simulink model "k1visbsp"  (Simulink 8.8)
settings: Solver=ode45  StartTime=0.0  StopTime=10.0  RelTol=1e-3  EnableMultiTasking=on
libraries: cdsIPCx x16, cdsEpicsOut x7, cdsBit2Word x6, cdsEpicsBinIn x3, cdsWord2Bit x3, cdsCDI64 x3, cdsCDO64 x3, TYPEB_MASTER x2, dac x2, cdsAdcx0 x1, cdsParameters x1
settings Model: SuppressorTable=22 serialization::archive 11 0 3 0 0 0 11 0  Creator=controls  LastModifiedBy=controls
settings DataIOCC: SignalLoggingSaveFormat=Dataset
settings DebuggingCC: UnderspecifiedInitializationDetection=Simplified  MergeDetectMultiDrivingBlocksExec=error  FcnCallInpInsideContextMsg=error  AllowSymbolicDim=off  StateNameClashWarn=none
settings GRTTargetCC: CombineOutputUpdateFcns=on  GRTInterface=off

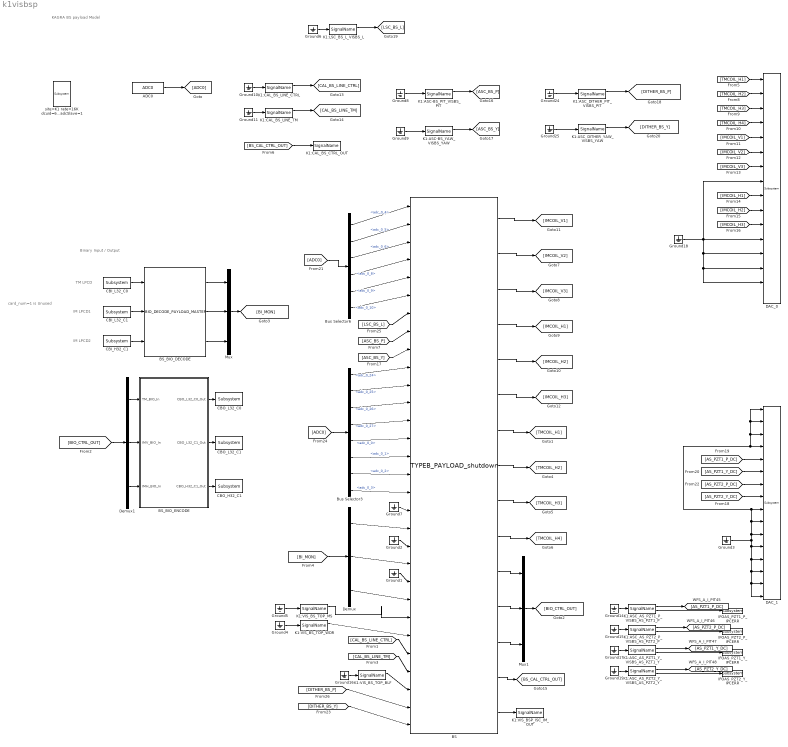
== system k1visbsp ==
  note: KAGRA BS payload Model
  note: TM LPCD
  note: Binary Input / Output
  note: card_num=1 is Unused
  note: IM LPCD1
  note: IM LPCD2
  ADC0 : cdsAdcx0/ADC0  Tag=cdsAdc  Description=|
      | type-GSC_16AI64SSA
      | card_num=0
      settings: AttributesFormatString=%<Description>\n%<Tag>
  BS : TYPEB_MASTER/TYPEB_PAYLOAD_shutdown
  BS_BIO_DECODE : TYPEB_MASTER/BIO_DECODE_PAYLOAD_MASTER
  BS_BIO_ENCODE : Subsystem  AncestorBlock=TYPEB_MASTER/BIO_ENCODE_PAYLOAD_MASTER
  Bus Selector3 : BusSelector  Description=ADC Selector  OutputSignals=adc_0_24,adc_0_25,adc_0_26,adc_0_27,adc_0_0,adc_0_1,adc_0_2,adc_0_3
      settings: AttributesFormatString=%<Description>
  Bus Selector6 : BusSelector  Description=ADC Selector  OutputSignals=adc_0_4,adc_0_5,adc_0_6,adc_0_8,adc_0_9,adc_0_10
      settings: AttributesFormatString=%<Description>
  CBI_H32_C1 : cdsCDI64/Subsystem  Tag=cdsCDI64  Description=card_num=3
      settings: AttributesFormatString=%<Tag>\n%<Description>
  CBI_L32_C0 : cdsCDI64/Subsystem  Tag=cdsCDI64  Description=card_num=0
      settings: AttributesFormatString=%<Tag>\n%<Description>
  CBI_L32_C1 : cdsCDI64/Subsystem  Tag=cdsCDI64  Description=card_num=2
      settings: AttributesFormatString=%<Tag>\n%<Description>
  CBO_H32_C1 : cdsCDO64/Subsystem  Tag=cdsCDO64  Description=card_num=3
      settings: AttributesFormatString=%<Tag>\n%<Description>
  CBO_L32_C0 : cdsCDO64/Subsystem  Tag=cdsCDO64  Description=card_num=0
      settings: AttributesFormatString=%<Tag>\n%<Description>
  CBO_L32_C1 : cdsCDO64/Subsystem  Tag=cdsCDO64  Description=card_num=2
      settings: AttributesFormatString=%<Tag>\n%<Description>
  DAC_0 : dac/Subsystem  Description=|
      | type=GSC_16AO16,
      | card_num=0
      settings: AttributesFormatString=%<Description>
  DAC_1 : dac/Subsystem  Description=|
      | type=GSC_16AO16,
      | card_num=1
      settings: AttributesFormatString=%<Description>
  Demux : Demux  Outputs=3
  Demux1 : Demux  Outputs=3
  Ground{1..11,14..19,24..25} (19 alike) : Ground
  IFOAS_PZT1_P_IPCERR : cdsEpicsOut/Subsystem  Tag=cdsEpicsOutput  Description=|
      | Purpose:                                          
      | Output a FE signal to an EPICS channel.           
      |                                                   
      | Operation:                                        
      | Takes input value and passes it to EPICS record.  
      |                                                   
      | Usage:                                            
      | Name the part with the desired EPICS rrecord name.
      settings: AttributesFormatString=%<Tag>
  IFOAS_PZT1_Y_IPCERR : cdsEpicsOut/Subsystem  Tag=cdsEpicsOutput  Description=|
      | Purpose:                                          
      | Output a FE signal to an EPICS channel.           
      |                                                   
      | Operation:                                        
      | Takes input value and passes it to EPICS record.  
      |                                                   
      | Usage:                                            
      | Name the part with the desired EPICS rrecord name.
      settings: AttributesFormatString=%<Tag>
  IFOAS_PZT2_P_IPCERR : cdsEpicsOut/Subsystem  Tag=cdsEpicsOutput  Description=|
      | Purpose:                                          
      | Output a FE signal to an EPICS channel.           
      |                                                   
      | Operation:                                        
      | Takes input value and passes it to EPICS record.  
      |                                                   
      | Usage:                                            
      | Name the part with the desired EPICS rrecord name.
      settings: AttributesFormatString=%<Tag>
  IFOAS_PZT2_Y_IPCERR : cdsEpicsOut/Subsystem  Tag=cdsEpicsOutput  Description=|
      | Purpose:                                          
      | Output a FE signal to an EPICS channel.           
      |                                                   
      | Operation:                                        
      | Takes input value and passes it to EPICS record.  
      |                                                   
      | Usage:                                            
      | Name the part with the desired EPICS rrecord name.
      settings: AttributesFormatString=%<Tag>
  K1:ASC-BS_PIT_VISBS_PIT : cdsIPCx/SignalName  Tag=cdsIPCx_PCIE  Description=Inter-Process Communication via PCI Express network.
      settings: AttributesFormatString=%<Tag>
  K1:ASC-BS_YAW_VISBS_YAW : cdsIPCx/SignalName  Tag=cdsIPCx_PCIE  Description=Inter-Process Communication via PCI Express network.
      settings: AttributesFormatString=%<Tag>
  K1:ASC_AS_PZT1_P_VISBS_AS_PZT1_P : cdsIPCx/SignalName  Tag=cdsIPCx_PCIE  Description=Inter-Process Communication via PCI Express network.
      settings: AttributesFormatString=%<Tag>
  K1:ASC_AS_PZT1_Y_VISBS_AS_PZT1_Y : cdsIPCx/SignalName  Tag=cdsIPCx_PCIE  Description=Inter-Process Communication via PCI Express network.
      settings: AttributesFormatString=%<Tag>
  K1:ASC_AS_PZT2_P_VISBS_AS_PZT2_P : cdsIPCx/SignalName  Tag=cdsIPCx_PCIE  Description=Inter-Process Communication via PCI Express network.
      settings: AttributesFormatString=%<Tag>
  K1:ASC_AS_PZT2_Y_VISBS_AS_PZT2_Y : cdsIPCx/SignalName  Tag=cdsIPCx_PCIE  Description=Inter-Process Communication via PCI Express network.
      settings: AttributesFormatString=%<Tag>
  K1:ASC_DITHER_PIT_VISBS_PIT : cdsIPCx/SignalName  Tag=cdsIPCx_PCIE  Description=Inter-Process Communication via PCI Express network.
      settings: AttributesFormatString=%<Tag>
  K1:ASC_DITHER_YAW_VISBS_YAW : cdsIPCx/SignalName  Tag=cdsIPCx_PCIE  Description=Inter-Process Communication via PCI Express network.
      settings: AttributesFormatString=%<Tag>
  K1:CAL_BS_CTRL_OUT : cdsIPCx/SignalName  Tag=cdsIPCx_PCIE  Description=Inter-Process Communication via PCI Express network.
      settings: AttributesFormatString=%<Tag>
  K1:CAL_BS_LINE_CTRL : cdsIPCx/SignalName  Tag=cdsIPCx_PCIE  Description=Inter-Process Communication via PCI Express network.
      settings: AttributesFormatString=%<Tag>
  K1:CAL_BS_LINE_TM : cdsIPCx/SignalName  Tag=cdsIPCx_PCIE  Description=Inter-Process Communication via PCI Express network.
      settings: AttributesFormatString=%<Tag>
  K1:LSC_BS_L_VISBS_L : cdsIPCx/SignalName  Tag=cdsIPCx_PCIE  Description=Inter-Process Communication via PCI Express network.
      settings: AttributesFormatString=%<Tag>
  K1:VIS_BSP_ISC_IM_OUT : cdsIPCx/SignalName  Tag=cdsIPCx_SHMEM  Description=Inter-Process Communication via Shared memory.
      settings: AttributesFormatString=%<Tag>
  K1:VIS_BS_TOP_BLF : cdsIPCx/SignalName  Tag=cdsIPCx_SHMEM  Description=Inter-Process Communication via Shared memory.
      settings: AttributesFormatString=%<Tag>
  K1:VIS_BS_TOP_MS : cdsIPCx/SignalName  Tag=cdsIPCx_SHMEM  Description=Inter-Process Communication via Shared memory.
      settings: AttributesFormatString=%<Tag>
  K1:VIS_BS_TOP_WDR : cdsIPCx/SignalName  Tag=cdsIPCx_SHMEM  Description=Inter-Process Communication via Shared memory.
      settings: AttributesFormatString=%<Tag>
  Mux : Mux  Inputs=3
  Mux1 : Mux  Inputs=3
  site=K1 rate=16K dcuid=61 host=k1bs specific_cpu=3 adcSlave=1 : cdsParameters/Subsystem  Tag=cdsParameters  Description=|
      | Purpose:                                                                                                                                                                                                                                
      | Provide system parameters to the FE code generator to properly configure the generated EPICS names, rep rate of the FE controller, and the Data Acquisition node ID for proper storage of data from this FE controller.                 
      |                                                                                                                                                                                                                                         
      | Useage:                                                                                                                                                                                                                                 
      | The part NAME field is used to identify the FE parameters. It must be of the form:                                                                                                                                                      
      | site=                                                                                                                                                                                                                                   
      | rate=                                                                                                                                                                                                                                   
      | dcuid=                                                                                                                                                                                                                                  
      |                                                                                                                                                                                                                                         
      | Where:                                                                                                                                                                                                                                  
      | site= argument may be H1, H2, L1, M1, G1, either as a single argument or multiple, for example site=H1,H2. These are the only names allowed. These will become the first two characters of all EPICS and signal names (for example G1:).
      |                                                                                                                                                                                                                                         
      | rate= may be 2K, 16K, 32K, or 64K                                                                                                                                                                                                       
      |                                                                                                                                                                                                                                         
      | dcuid= is site specific ie it must be unique at each site.
      settings: AttributesFormatString=%<Tag>
  wires:
  ADC0/1 -> [ADC0]
  [ADC0] -> Bus Selector6/1
  BS/10 -> [TMCOIL_H4]
  BS/9 -> [TMCOIL_H3]
  BS/8 -> [TMCOIL_H2]
  BS/7 -> [TMCOIL_H1]
  BS/1 -> [IMCOIL_V1]
  BS/2 -> [IMCOIL_V2]
  BS/3 -> [IMCOIL_V3]
  BS/4 -> [IMCOIL_H1]
  BS/5 -> [IMCOIL_H2]
  BS/6 -> [IMCOIL_H3]
  Ground18/1 -> DAC_0/12, DAC_0/13, DAC_0/14, DAC_0/15, DAC_0/8
  Bus Selector6/1 -> BS/1  "<adc_0_4>"
  Bus Selector6/2 -> BS/2  "<adc_0_5>"
  Bus Selector6/3 -> BS/3  "<adc_0_6>"
  [TMCOIL_H2] -> DAC_0/2
  [TMCOIL_H3] -> DAC_0/3
  [TMCOIL_H1] -> DAC_0/1
  [TMCOIL_H4] -> DAC_0/4
  [IMCOIL_V1] -> DAC_0/5
  [IMCOIL_V2] -> DAC_0/6
  [IMCOIL_V3] -> DAC_0/7
  Bus Selector6/4 -> BS/4  "<adc_0_8>"
  Bus Selector6/5 -> BS/5  "<adc_0_9>"
  Bus Selector6/6 -> BS/6  "<adc_0_10>"
  [IMCOIL_H3] -> DAC_0/11
  [IMCOIL_H2] -> DAC_0/10
  [IMCOIL_H1] -> DAC_0/9
  [LSC_BS_L] -> BS/7
  [ADC0] -> Bus Selector3/1
  Bus Selector3/1 -> BS/10  "<adc_0_24>"
  Bus Selector3/2 -> BS/11  "<adc_0_25>"
  Bus Selector3/3 -> BS/12  "<adc_0_26>"
  Bus Selector3/4 -> BS/13  "<adc_0_27>"
  BS_BIO_ENCODE/3(CBO_H32_C1_Out) -> CBO_H32_C1/1
  BS_BIO_ENCODE/2(CBO_L32_C1_Out) -> CBO_L32_C1/1
  CBI_L32_C1/1 -> BS_BIO_DECODE/2
  CBI_H32_C1/1 -> BS_BIO_DECODE/3
  BS_BIO_DECODE/2 -> Mux/2
  BS_BIO_DECODE/3 -> Mux/3
  BS_BIO_DECODE/1 -> Mux/1
  Mux/1 -> [BI_MON]
  Demux1/2 -> BS_BIO_ENCODE/2(IMV_BIO_In)
  Demux1/3 -> BS_BIO_ENCODE/3(IMH_BIO_In)
  Demux1/1 -> BS_BIO_ENCODE/1(TM_BIO_In)
  [BIO_CTRL_OUT] -> Demux1/1
  Mux1/1 -> [BIO_CTRL_OUT]
  [BI_MON] -> Demux/1
  Demux/1 -> BS/19
  Demux/2 -> BS/21
  Demux/3 -> BS/23
  Ground7/1 -> BS/18
  Ground1/1 -> BS/22
  Ground2/1 -> BS/20
  Ground4/1 -> K1:VIS_BS_TOP_WDR/1
  Ground5/1 -> K1:VIS_BS_TOP_MS/1
  K1:VIS_BS_TOP_WDR/1 -> BS/25
  K1:VIS_BS_TOP_MS/1 -> BS/24
  Ground10/1 -> K1:CAL_BS_LINE_CTRL/1
  K1:CAL_BS_LINE_CTRL/1 -> [CAL_BS_LINE_CTRL]
  Ground11/1 -> K1:CAL_BS_LINE_TM/1
  K1:CAL_BS_LINE_TM/1 -> [CAL_BS_LINE_TM]
  [CAL_BS_LINE_CTRL] -> BS/26
  [CAL_BS_LINE_TM] -> BS/27
  BS/14 -> [BS_CAL_CTRL_OUT]
  [BS_CAL_CTRL_OUT] -> K1:CAL_BS_CTRL_OUT/1
  Ground3/1 -> DAC_1/13, DAC_1/14, DAC_1/15, DAC_1/16, DAC_1/12, DAC_1/1, DAC_1/2, DAC_1/3, DAC_1/4, DAC_1/9, DAC_1/10, DAC_1/11
  Bus Selector3/5 -> BS/14  "<adc_0_0>"
  Bus Selector3/6 -> BS/15  "<adc_0_1>"
  Bus Selector3/7 -> BS/16  "<adc_0_2>"
  Bus Selector3/8 -> BS/17  "<adc_0_3>"
  [ASC_BS_P] -> BS/8
  [ASC_BS_Y] -> BS/9
  Ground16/1 -> K1:VIS_BS_TOP_BLF/1
  K1:VIS_BS_TOP_BLF/1 -> BS/28
  BS/11 -> Mux1/1
  BS/12 -> Mux1/2
  BS/13 -> Mux1/3
  [DITHER_BS_Y] -> BS/30
  K1:ASC_AS_PZT1_P_VISBS_AS_PZT1_P/2 -> IFOAS_PZT1_P_IPCERR/1
  K1:ASC_AS_PZT2_P_VISBS_AS_PZT2_P/2 -> IFOAS_PZT2_P_IPCERR/1
  K1:ASC_AS_PZT1_Y_VISBS_AS_PZT1_Y/2 -> IFOAS_PZT1_Y_IPCERR/1
  K1:ASC_AS_PZT2_Y_VISBS_AS_PZT2_Y/2 -> IFOAS_PZT2_Y_IPCERR/1
  K1:ASC_AS_PZT1_P_VISBS_AS_PZT1_P/1 -> [AS_PZT1_P_DC]
  K1:ASC_AS_PZT2_P_VISBS_AS_PZT2_P/1 -> [AS_PZT2_P_DC]
  K1:ASC_AS_PZT1_Y_VISBS_AS_PZT1_Y/1 -> [AS_PZT1_Y_DC]
  K1:ASC_AS_PZT2_Y_VISBS_AS_PZT2_Y/1 -> [AS_PZT2_Y_DC]
  Ground14/1 -> K1:ASC_AS_PZT1_P_VISBS_AS_PZT1_P/1
  Ground15/1 -> K1:ASC_AS_PZT2_P_VISBS_AS_PZT2_P/1
  Ground17/1 -> K1:ASC_AS_PZT1_Y_VISBS_AS_PZT1_Y/1
  Ground19/1 -> K1:ASC_AS_PZT2_Y_VISBS_AS_PZT2_Y/1
  [AS_PZT2_Y_DC] -> DAC_1/8
  [AS_PZT2_P_DC] -> DAC_1/7
  [AS_PZT1_Y_DC] -> DAC_1/6
  [AS_PZT1_P_DC] -> DAC_1/5
  Ground6/1 -> K1:LSC_BS_L_VISBS_L/1
  K1:LSC_BS_L_VISBS_L/1 -> [LSC_BS_L]
  Ground8/1 -> K1:ASC-BS_PIT_VISBS_PIT/1
  Ground9/1 -> K1:ASC-BS_YAW_VISBS_YAW/1
  Ground25/1 -> K1:ASC_DITHER_YAW_VISBS_YAW/1
  Ground24/1 -> K1:ASC_DITHER_PIT_VISBS_PIT/1
  [DITHER_BS_P] -> BS/29
  K1:ASC-BS_PIT_VISBS_PIT/1 -> [ASC_BS_P]
  K1:ASC-BS_YAW_VISBS_YAW/1 -> [ASC_BS_Y]
  K1:ASC_DITHER_PIT_VISBS_PIT/1 -> [DITHER_BS_P]
  K1:ASC_DITHER_YAW_VISBS_YAW/1 -> [DITHER_BS_Y]
  BS_BIO_ENCODE/1(CBO_L32_C0_Out) -> CBO_L32_C0/1
  CBI_L32_C0/1 -> BS_BIO_DECODE/1
  BS/15 -> K1:VIS_BSP_ISC_IM_OUT/1

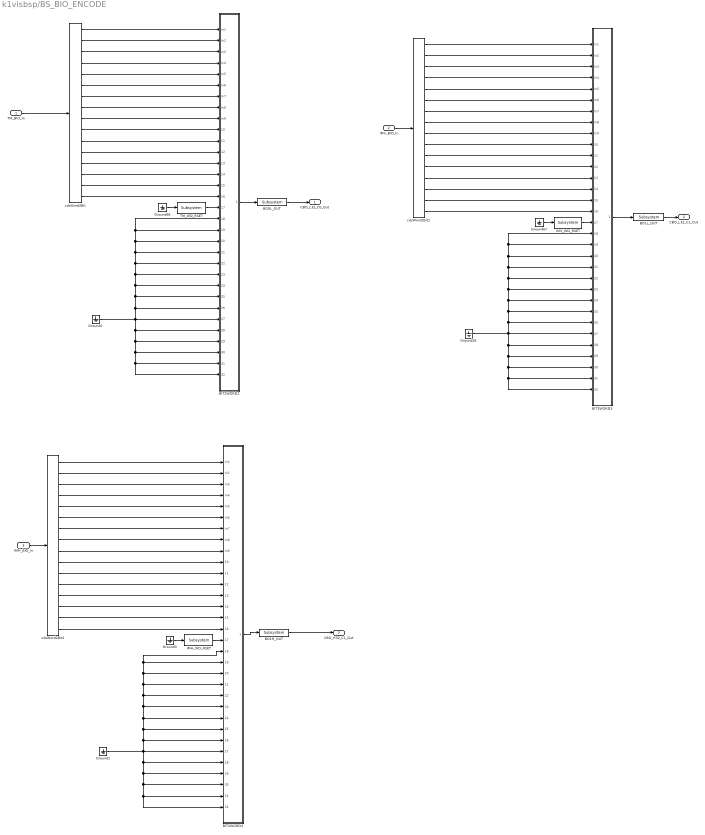
== system k1visbsp/BS_BIO_ENCODE ==
  TM_BIO_In : Inport
  IMV_BIO_In : Inport  Port=2
  IMH_BIO_In : Inport  Port=3
  BIT2WORD2 : Subsystem
  BIT2WORD3 : Subsystem
  BIT2WORD4 : Subsystem
  BO0L_OUT : cdsEpicsOut/Subsystem  Tag=cdsEpicsOutput  Description=|
      | Purpose:                                          
      | Output a FE signal to an EPICS channel.           
      |                                                   
      | Operation:                                        
      | Takes input value and passes it to EPICS record.  
      |                                                   
      | Usage:                                            
      | Name the part with the desired EPICS rrecord name.
      settings: AttributesFormatString=%<Tag>
  BO1H_OUT : cdsEpicsOut/Subsystem  Tag=cdsEpicsOutput  Description=|
      | Purpose:                                          
      | Output a FE signal to an EPICS channel.           
      |                                                   
      | Operation:                                        
      | Takes input value and passes it to EPICS record.  
      |                                                   
      | Usage:                                            
      | Name the part with the desired EPICS rrecord name.
      settings: AttributesFormatString=%<Tag>
  BO1L_OUT : cdsEpicsOut/Subsystem  Tag=cdsEpicsOutput  Description=|
      | Purpose:                                          
      | Output a FE signal to an EPICS channel.           
      |                                                   
      | Operation:                                        
      | Takes input value and passes it to EPICS record.  
      |                                                   
      | Usage:                                            
      | Name the part with the desired EPICS rrecord name.
      settings: AttributesFormatString=%<Tag>
  Ground{1..3,26,66..67} (6 alike) : Ground
  IMH_WD_RSET : cdsEpicsBinIn/Subsystem  Tag=cdsEpicsBinIn  Description=|
      | Purpose:                                                                            
      | Create an EPICS binary (0 or 1) input channel to the FE realtime controls.          
      |                                                                                     
      | Operation:                                                                          
      | Outputs value from an EPICS ai record. Value is binary input (bi Epics record type).
      |                                                                                     
      | Usage:                                                                              
      | Name the part with the desired EPICS channel name.
      settings: AttributesFormatString=%<Tag>
  IMV_WD_RSET : cdsEpicsBinIn/Subsystem  Tag=cdsEpicsBinIn  Description=|
      | Purpose:                                                                            
      | Create an EPICS binary (0 or 1) input channel to the FE realtime controls.          
      |                                                                                     
      | Operation:                                                                          
      | Outputs value from an EPICS ai record. Value is binary input (bi Epics record type).
      |                                                                                     
      | Usage:                                                                              
      | Name the part with the desired EPICS channel name.
      settings: AttributesFormatString=%<Tag>
  TM_WD_RSET : cdsEpicsBinIn/Subsystem  Tag=cdsEpicsBinIn  Description=|
      | Purpose:                                                                            
      | Create an EPICS binary (0 or 1) input channel to the FE realtime controls.          
      |                                                                                     
      | Operation:                                                                          
      | Outputs value from an EPICS ai record. Value is binary input (bi Epics record type).
      |                                                                                     
      | Usage:                                                                              
      | Name the part with the desired EPICS channel name.
      settings: AttributesFormatString=%<Tag>
  cdsWord2Bit : cdsWord2Bit/cdsWord2Bit  Tag=cdsWord2Bit  Description=Generate 16 0/1 outputs from single 16-bit integer input
      settings: AttributesFormatString=cdsWord2Bit
  cdsWord2Bit1 : cdsWord2Bit/cdsWord2Bit  Tag=cdsWord2Bit  Description=Generate 16 0/1 outputs from single 16-bit integer input
      settings: AttributesFormatString=cdsWord2Bit
  cdsWord2Bit2 : cdsWord2Bit/cdsWord2Bit  Tag=cdsWord2Bit  Description=Generate 16 0/1 outputs from single 16-bit integer input
      settings: AttributesFormatString=cdsWord2Bit
  CBO_L32_C0_Out : Outport
  CBO_L32_C1_Out : Outport  Port=2
  CBO_H32_C1_Out : Outport  Port=3
  wires:
  cdsWord2Bit2/16 -> BIT2WORD4/16(In16)
  cdsWord2Bit2/12 -> BIT2WORD4/12(In12)
  cdsWord2Bit2/14 -> BIT2WORD4/14(In14)
  cdsWord2Bit2/15 -> BIT2WORD4/15(In15)
  cdsWord2Bit2/13 -> BIT2WORD4/13(In13)
  cdsWord2Bit1/13 -> BIT2WORD3/13(In13)
  cdsWord2Bit1/15 -> BIT2WORD3/15(In15)
  cdsWord2Bit1/14 -> BIT2WORD3/14(In14)
  cdsWord2Bit1/16 -> BIT2WORD3/16(In16)
  cdsWord2Bit1/12 -> BIT2WORD3/12(In12)
  cdsWord2Bit/16 -> BIT2WORD2/16(In16)
  cdsWord2Bit/15 -> BIT2WORD2/15(In15)
  cdsWord2Bit/14 -> BIT2WORD2/14(In14)
  cdsWord2Bit/13 -> BIT2WORD2/13(In13)
  cdsWord2Bit/12 -> BIT2WORD2/12(In12)
  IMH_WD_RSET/1 -> BIT2WORD4/17(In17)
  Ground3/1 -> IMH_WD_RSET/1
  cdsWord2Bit2/11 -> BIT2WORD4/11(In11)
  cdsWord2Bit2/10 -> BIT2WORD4/10(In10)
  cdsWord2Bit2/9 -> BIT2WORD4/9(In9)
  cdsWord2Bit2/8 -> BIT2WORD4/8(In8)
  cdsWord2Bit2/7 -> BIT2WORD4/7(In7)
  cdsWord2Bit2/1 -> BIT2WORD4/1(In1)
  cdsWord2Bit2/6 -> BIT2WORD4/6(In6)
  cdsWord2Bit2/2 -> BIT2WORD4/2(In2)
  cdsWord2Bit2/3 -> BIT2WORD4/3(In3)
  cdsWord2Bit2/5 -> BIT2WORD4/5(In5)
  cdsWord2Bit2/4 -> BIT2WORD4/4(In4)
  IMH_BIO_In/1 -> cdsWord2Bit2/1
  Ground1/1 -> BIT2WORD4/31(In31), BIT2WORD4/32(In32), BIT2WORD4/30(In30), BIT2WORD4/29(In29), BIT2WORD4/28(In28), BIT2WORD4/18(In18), BIT2WORD4/19(In19), BIT2WORD4/20(In20), BIT2WORD4/21(In21), BIT2WORD4/22(In22), BIT2WORD4/23(In23), BIT2WORD4/24(In24), BIT2WORD4/25(In25), BIT2WORD4/26(In26), BIT2WORD4/27(In27)
  BIT2WORD4/1(Out1) -> BO1H_OUT/1
  BO1L_OUT/1 -> CBO_L32_C1_Out/1
  BIT2WORD3/1(Out1) -> BO1L_OUT/1
  BIT2WORD2/1(Out1) -> BO0L_OUT/1
  BO1H_OUT/1 -> CBO_H32_C1_Out/1
  BO0L_OUT/1 -> CBO_L32_C0_Out/1
  IMV_WD_RSET/1 -> BIT2WORD3/17(In17)
  TM_WD_RSET/1 -> BIT2WORD2/17(In17)
  Ground67/1 -> IMV_WD_RSET/1
  Ground66/1 -> TM_WD_RSET/1
  cdsWord2Bit1/11 -> BIT2WORD3/11(In11)
  cdsWord2Bit1/10 -> BIT2WORD3/10(In10)
  cdsWord2Bit1/9 -> BIT2WORD3/9(In9)
  cdsWord2Bit1/8 -> BIT2WORD3/8(In8)
  cdsWord2Bit1/7 -> BIT2WORD3/7(In7)
  cdsWord2Bit1/1 -> BIT2WORD3/1(In1)
  cdsWord2Bit1/6 -> BIT2WORD3/6(In6)
  cdsWord2Bit1/2 -> BIT2WORD3/2(In2)
  cdsWord2Bit1/3 -> BIT2WORD3/3(In3)
  cdsWord2Bit1/5 -> BIT2WORD3/5(In5)
  cdsWord2Bit1/4 -> BIT2WORD3/4(In4)
  IMV_BIO_In/1 -> cdsWord2Bit1/1
  Ground26/1 -> BIT2WORD3/27(In27), BIT2WORD3/29(In29), BIT2WORD3/30(In30), BIT2WORD3/32(In32), BIT2WORD3/31(In31), BIT2WORD3/28(In28), BIT2WORD3/26(In26), BIT2WORD3/25(In25), BIT2WORD3/24(In24), BIT2WORD3/23(In23), BIT2WORD3/22(In22), BIT2WORD3/21(In21), BIT2WORD3/19(In19), BIT2WORD3/18(In18), BIT2WORD3/20(In20)
  cdsWord2Bit/11 -> BIT2WORD2/11(In11)
  cdsWord2Bit/10 -> BIT2WORD2/10(In10)
  cdsWord2Bit/9 -> BIT2WORD2/9(In9)
  cdsWord2Bit/8 -> BIT2WORD2/8(In8)
  cdsWord2Bit/7 -> BIT2WORD2/7(In7)
  cdsWord2Bit/1 -> BIT2WORD2/1(In1)
  cdsWord2Bit/2 -> BIT2WORD2/2(In2)
  cdsWord2Bit/3 -> BIT2WORD2/3(In3)
  cdsWord2Bit/4 -> BIT2WORD2/4(In4)
  TM_BIO_In/1 -> cdsWord2Bit/1
  Ground2/1 -> BIT2WORD2/27(In27), BIT2WORD2/29(In29), BIT2WORD2/30(In30), BIT2WORD2/32(In32), BIT2WORD2/31(In31), BIT2WORD2/28(In28), BIT2WORD2/26(In26), BIT2WORD2/25(In25), BIT2WORD2/24(In24), BIT2WORD2/23(In23), BIT2WORD2/22(In22), BIT2WORD2/21(In21), BIT2WORD2/19(In19), BIT2WORD2/18(In18), BIT2WORD2/20(In20)
  cdsWord2Bit/6 -> BIT2WORD2/6(In6)
  cdsWord2Bit/5 -> BIT2WORD2/5(In5)

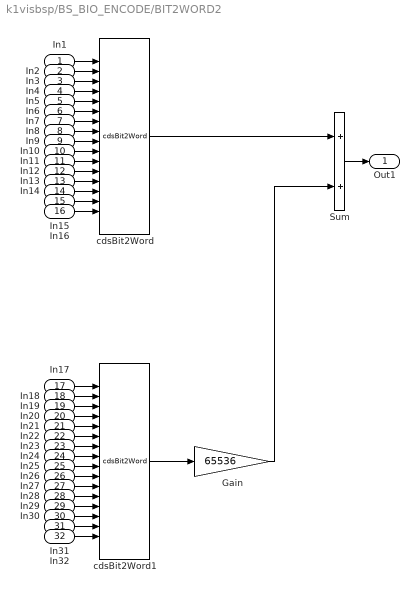
== system k1visbsp/BS_BIO_ENCODE/BIT2WORD2 ==
  In1 : Inport
  In2 : Inport  Port=2
  In3 : Inport  Port=3
  In4 : Inport  Port=4
  In5 : Inport  Port=5
  In6 : Inport  Port=6
  In7 : Inport  Port=7
  In8 : Inport  Port=8
  In9 : Inport  Port=9
  In10 : Inport  Port=10
  In11 : Inport  Port=11
  In12 : Inport  Port=12
  In13 : Inport  Port=13
  In14 : Inport  Port=14
  In15 : Inport  Port=15
  In16 : Inport  Port=16
  In17 : Inport  Port=17
  In18 : Inport  Port=18
  In19 : Inport  Port=19
  In20 : Inport  Port=20
  In21 : Inport  Port=21
  In22 : Inport  Port=22
  In23 : Inport  Port=23
  In24 : Inport  Port=24
  In25 : Inport  Port=25
  In26 : Inport  Port=26
  In27 : Inport  Port=27
  In28 : Inport  Port=28
  In29 : Inport  Port=29
  In30 : Inport  Port=30
  In31 : Inport  Port=31
  In32 : Inport  Port=32
  Gain : Gain  Gain=65536
  Sum : Sum
  cdsBit2Word : cdsBit2Word/cdsBit2Word  Tag=cdsBit2Word  Description=Forms single 16 bit integer from 16 0/1 inputs.
      settings: AttributesFormatString=%<Tag>
  cdsBit2Word1 : cdsBit2Word/cdsBit2Word  Tag=cdsBit2Word  Description=Forms single 16 bit integer from 16 0/1 inputs.
      settings: AttributesFormatString=%<Tag>
  Out1 : Outport
  wires:
  In32/1 -> cdsBit2Word1/16
  In31/1 -> cdsBit2Word1/15
  In30/1 -> cdsBit2Word1/14
  In29/1 -> cdsBit2Word1/13
  In28/1 -> cdsBit2Word1/12
  In27/1 -> cdsBit2Word1/11
  In26/1 -> cdsBit2Word1/10
  In25/1 -> cdsBit2Word1/9
  In24/1 -> cdsBit2Word1/8
  In23/1 -> cdsBit2Word1/7
  In22/1 -> cdsBit2Word1/6
  In21/1 -> cdsBit2Word1/5
  In20/1 -> cdsBit2Word1/4
  In19/1 -> cdsBit2Word1/3
  In18/1 -> cdsBit2Word1/2
  In17/1 -> cdsBit2Word1/1
  In16/1 -> cdsBit2Word/16
  In15/1 -> cdsBit2Word/15
  In14/1 -> cdsBit2Word/14
  In13/1 -> cdsBit2Word/13
  In12/1 -> cdsBit2Word/12
  In11/1 -> cdsBit2Word/11
  Sum/1 -> Out1/1
  In10/1 -> cdsBit2Word/10
  In9/1 -> cdsBit2Word/9
  In8/1 -> cdsBit2Word/8
  In7/1 -> cdsBit2Word/7
  In6/1 -> cdsBit2Word/6
  In5/1 -> cdsBit2Word/5
  In4/1 -> cdsBit2Word/4
  In3/1 -> cdsBit2Word/3
  In2/1 -> cdsBit2Word/2
  In1/1 -> cdsBit2Word/1
  cdsBit2Word/1 -> Sum/1
  cdsBit2Word1/1 -> Gain/1
  Gain/1 -> Sum/2

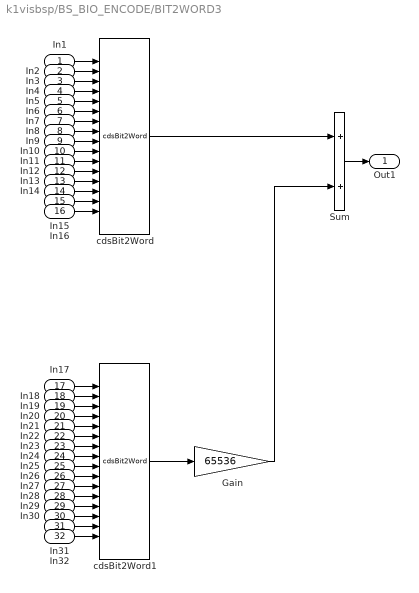
== system k1visbsp/BS_BIO_ENCODE/BIT2WORD3 ==
  In1 : Inport
  In2 : Inport  Port=2
  In3 : Inport  Port=3
  In4 : Inport  Port=4
  In5 : Inport  Port=5
  In6 : Inport  Port=6
  In7 : Inport  Port=7
  In8 : Inport  Port=8
  In9 : Inport  Port=9
  In10 : Inport  Port=10
  In11 : Inport  Port=11
  In12 : Inport  Port=12
  In13 : Inport  Port=13
  In14 : Inport  Port=14
  In15 : Inport  Port=15
  In16 : Inport  Port=16
  In17 : Inport  Port=17
  In18 : Inport  Port=18
  In19 : Inport  Port=19
  In20 : Inport  Port=20
  In21 : Inport  Port=21
  In22 : Inport  Port=22
  In23 : Inport  Port=23
  In24 : Inport  Port=24
  In25 : Inport  Port=25
  In26 : Inport  Port=26
  In27 : Inport  Port=27
  In28 : Inport  Port=28
  In29 : Inport  Port=29
  In30 : Inport  Port=30
  In31 : Inport  Port=31
  In32 : Inport  Port=32
  Gain : Gain  Gain=65536
  Sum : Sum
  cdsBit2Word : cdsBit2Word/cdsBit2Word  Tag=cdsBit2Word  Description=Forms single 16 bit integer from 16 0/1 inputs.
      settings: AttributesFormatString=%<Tag>
  cdsBit2Word1 : cdsBit2Word/cdsBit2Word  Tag=cdsBit2Word  Description=Forms single 16 bit integer from 16 0/1 inputs.
      settings: AttributesFormatString=%<Tag>
  Out1 : Outport
  wires:
  In32/1 -> cdsBit2Word1/16
  In31/1 -> cdsBit2Word1/15
  In30/1 -> cdsBit2Word1/14
  In29/1 -> cdsBit2Word1/13
  In28/1 -> cdsBit2Word1/12
  In27/1 -> cdsBit2Word1/11
  In26/1 -> cdsBit2Word1/10
  In25/1 -> cdsBit2Word1/9
  In24/1 -> cdsBit2Word1/8
  In23/1 -> cdsBit2Word1/7
  In22/1 -> cdsBit2Word1/6
  In21/1 -> cdsBit2Word1/5
  In20/1 -> cdsBit2Word1/4
  In19/1 -> cdsBit2Word1/3
  In18/1 -> cdsBit2Word1/2
  In17/1 -> cdsBit2Word1/1
  In16/1 -> cdsBit2Word/16
  In15/1 -> cdsBit2Word/15
  In14/1 -> cdsBit2Word/14
  In13/1 -> cdsBit2Word/13
  In12/1 -> cdsBit2Word/12
  In11/1 -> cdsBit2Word/11
  Sum/1 -> Out1/1
  In10/1 -> cdsBit2Word/10
  In9/1 -> cdsBit2Word/9
  In8/1 -> cdsBit2Word/8
  In7/1 -> cdsBit2Word/7
  In6/1 -> cdsBit2Word/6
  In5/1 -> cdsBit2Word/5
  In4/1 -> cdsBit2Word/4
  In3/1 -> cdsBit2Word/3
  In2/1 -> cdsBit2Word/2
  In1/1 -> cdsBit2Word/1
  cdsBit2Word/1 -> Sum/1
  cdsBit2Word1/1 -> Gain/1
  Gain/1 -> Sum/2

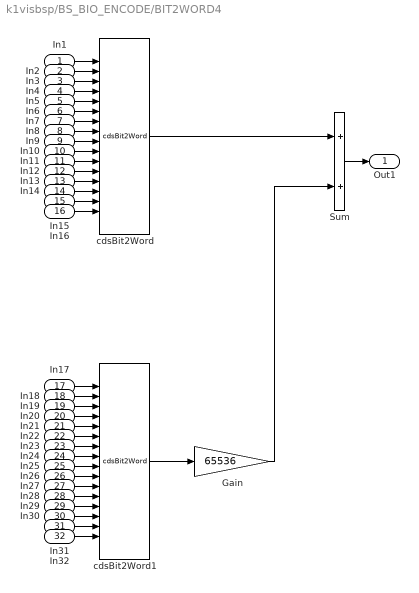
== system k1visbsp/BS_BIO_ENCODE/BIT2WORD4 ==
  In1 : Inport
  In2 : Inport  Port=2
  In3 : Inport  Port=3
  In4 : Inport  Port=4
  In5 : Inport  Port=5
  In6 : Inport  Port=6
  In7 : Inport  Port=7
  In8 : Inport  Port=8
  In9 : Inport  Port=9
  In10 : Inport  Port=10
  In11 : Inport  Port=11
  In12 : Inport  Port=12
  In13 : Inport  Port=13
  In14 : Inport  Port=14
  In15 : Inport  Port=15
  In16 : Inport  Port=16
  In17 : Inport  Port=17
  In18 : Inport  Port=18
  In19 : Inport  Port=19
  In20 : Inport  Port=20
  In21 : Inport  Port=21
  In22 : Inport  Port=22
  In23 : Inport  Port=23
  In24 : Inport  Port=24
  In25 : Inport  Port=25
  In26 : Inport  Port=26
  In27 : Inport  Port=27
  In28 : Inport  Port=28
  In29 : Inport  Port=29
  In30 : Inport  Port=30
  In31 : Inport  Port=31
  In32 : Inport  Port=32
  Gain : Gain  Gain=65536
  Sum : Sum
  cdsBit2Word : cdsBit2Word/cdsBit2Word  Tag=cdsBit2Word  Description=Forms single 16 bit integer from 16 0/1 inputs.
      settings: AttributesFormatString=%<Tag>
  cdsBit2Word1 : cdsBit2Word/cdsBit2Word  Tag=cdsBit2Word  Description=Forms single 16 bit integer from 16 0/1 inputs.
      settings: AttributesFormatString=%<Tag>
  Out1 : Outport
  wires:
  In32/1 -> cdsBit2Word1/16
  In31/1 -> cdsBit2Word1/15
  In30/1 -> cdsBit2Word1/14
  In29/1 -> cdsBit2Word1/13
  In28/1 -> cdsBit2Word1/12
  In27/1 -> cdsBit2Word1/11
  In26/1 -> cdsBit2Word1/10
  In25/1 -> cdsBit2Word1/9
  In24/1 -> cdsBit2Word1/8
  In23/1 -> cdsBit2Word1/7
  In22/1 -> cdsBit2Word1/6
  In21/1 -> cdsBit2Word1/5
  In20/1 -> cdsBit2Word1/4
  In19/1 -> cdsBit2Word1/3
  In18/1 -> cdsBit2Word1/2
  In17/1 -> cdsBit2Word1/1
  In16/1 -> cdsBit2Word/16
  In15/1 -> cdsBit2Word/15
  In14/1 -> cdsBit2Word/14
  In13/1 -> cdsBit2Word/13
  In12/1 -> cdsBit2Word/12
  In11/1 -> cdsBit2Word/11
  Sum/1 -> Out1/1
  In10/1 -> cdsBit2Word/10
  In9/1 -> cdsBit2Word/9
  In8/1 -> cdsBit2Word/8
  In7/1 -> cdsBit2Word/7
  In6/1 -> cdsBit2Word/6
  In5/1 -> cdsBit2Word/5
  In4/1 -> cdsBit2Word/4
  In3/1 -> cdsBit2Word/3
  In2/1 -> cdsBit2Word/2
  In1/1 -> cdsBit2Word/1
  cdsBit2Word/1 -> Sum/1
  cdsBit2Word1/1 -> Gain/1
  Gain/1 -> Sum/2
